simulink model "Practica1_4_4"  (R2015a)
settings: Solver=ode45  StartTime=0.0  StopTime=10.0  RelTol=1e-3
settings Model: Creator=redes  LastModifiedBy=redes

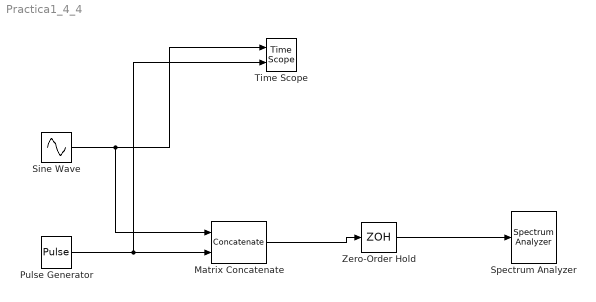
== system Practica1_4_4 ==
  Matrix Concatenate : Concatenate  Mode=Multidimensional array  ConcatenateDimension=2
  Pulse Generator : DiscretePulseGenerator  PulseType=Time based  Period=1  PulseWidth=50  PhaseDelay=0.0025
  Sine Wave : Sin  Frequency=2*pi*1  SampleTime=0.0025
  Spectrum Analyzer : SpectrumAnalyzer
  Time Scope : TimeScope  DefaultConfigurationName=spbscopes.TimeScopeBlockCfg  NumInputPorts=2
  Zero-Order Hold : ZeroOrderHold  SampleTime=0.0025
  wires:
  Sine Wave/1 -> Matrix Concatenate/1, Time Scope/1
  Pulse Generator/1 -> Time Scope/2, Matrix Concatenate/2
  Matrix Concatenate/1 -> Zero-Order Hold/1
  Zero-Order Hold/1 -> Spectrum Analyzer/1
